simulink model "Water_Supply_Network_AMONG_US"  (R2024a)
settings: Solver=VariableStepAuto  StartTime=0  StopTime=10  RelTol=1e3
model workspace (MAT data in the model file):
  a = [3 8 5 5 2 7 2 5]
  c = [100 100 100 100 100 100 100 100]
  c_init = [50 50 50 0 0 0 0 0]
  d = [2 0.5 4 3 4 5 7 4]
  f = [0.4 0.6 0.2 1 0.4 0.1 0.9 0.6]
  p = [15 20 5 7 3 5 5]
settings Model: Creator=Anna  LastModifiedBy=eveli

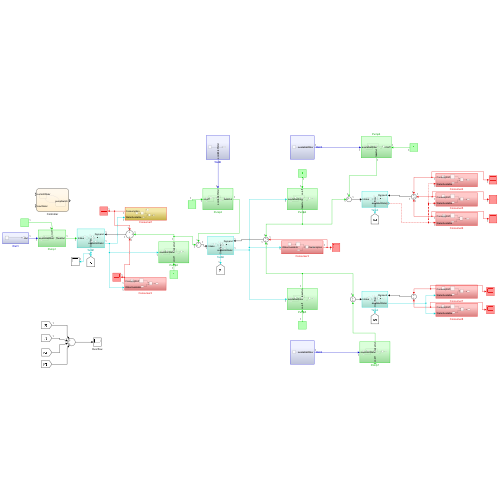
[thumbnail: Simulink's stored preview of the top-level diagram]
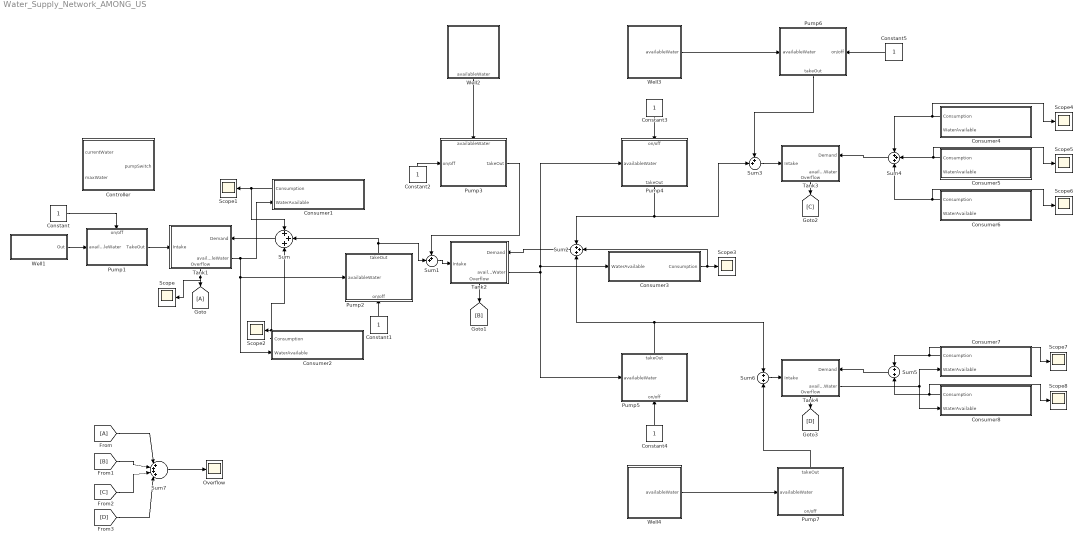
== system Water_Supply_Network_AMONG_US ==
  Constant{,1..5} (6 alike) : Constant  OutDataTypeStr=boolean
  Consumer1 : Subsystem
      settings: PortSchema="{\"entries\":[{\"content\":{\"sides\":[{\"content\":{\"connectorIds\":[\"Out1\",\"In1\"]},\"type\":\"ConnectorPlacement.EquallySpacedRectSide\",\"uuid\":\"64b5a97a-4244-4f26-899d-15714f2aa8f6\"},{\"content\":{\"side\":\"RIGHT\"},\"type\":\"ConnectorPlacement.EquallySpacedRectSide\",\"uuid\":\"d3b45f67-9c9d-4eef-86a5-95557b8542c4\"},{\"content\":{\"side\":\"TOP\"},\"type\":\"ConnectorPlacement.EquallySpacedRectSide\",\"uuid\":\"2b7281c0-f61f-45e3-808b-a4fd1d62cbbb\"}]},\"type\":\"ConnectorPlacement.EquallySpacedConnector\",\"uuid\":\"1937d4df-e955-4a14-a18e-eb0cc3956b4d\"}],\"packageUris\":[\"http://schema.mathworks.com/mf0/Connector/R2020b\"],\"version\":\"1.0\"}"
  Consumer2 : Subsystem
      settings: PortSchema="{\"entries\":[{\"content\":{\"sides\":[{\"content\":{\"connectorIds\":[\"Out1\",\"In1\"]},\"type\":\"ConnectorPlacement.EquallySpacedRectSide\",\"uuid\":\"64b5a97a-4244-4f26-899d-15714f2aa8f6\"},{\"content\":{\"side\":\"RIGHT\"},\"type\":\"ConnectorPlacement.EquallySpacedRectSide\",\"uuid\":\"d3b45f67-9c9d-4eef-86a5-95557b8542c4\"},{\"content\":{\"side\":\"TOP\"},\"type\":\"ConnectorPlacement.EquallySpacedRectSide\",\"uuid\":\"2b7281c0-f61f-45e3-808b-a4fd1d62cbbb\"}]},\"type\":\"ConnectorPlacement.EquallySpacedConnector\",\"uuid\":\"1937d4df-e955-4a14-a18e-eb0cc3956b4d\"}],\"packageUris\":[\"http://schema.mathworks.com/mf0/Connector/R2020b\"],\"version\":\"1.0\"}"
  Consumer3 : Subsystem
  Consumer4 : Subsystem
      settings: PortSchema="{\"entries\":[{\"content\":{\"sides\":[{\"content\":{\"connectorIds\":[\"Out1\",\"In1\"]},\"type\":\"ConnectorPlacement.EquallySpacedRectSide\",\"uuid\":\"64b5a97a-4244-4f26-899d-15714f2aa8f6\"},{\"content\":{\"side\":\"RIGHT\"},\"type\":\"ConnectorPlacement.EquallySpacedRectSide\",\"uuid\":\"d3b45f67-9c9d-4eef-86a5-95557b8542c4\"},{\"content\":{\"side\":\"TOP\"},\"type\":\"ConnectorPlacement.EquallySpacedRectSide\",\"uuid\":\"2b7281c0-f61f-45e3-808b-a4fd1d62cbbb\"}]},\"type\":\"ConnectorPlacement.EquallySpacedConnector\",\"uuid\":\"1937d4df-e955-4a14-a18e-eb0cc3956b4d\"}],\"packageUris\":[\"http://schema.mathworks.com/mf0/Connector/R2020b\"],\"version\":\"1.0\"}"
  Consumer5 : Subsystem
      settings: PortSchema="{\"entries\":[{\"content\":{\"sides\":[{\"content\":{\"connectorIds\":[\"Out1\",\"In1\"]},\"type\":\"ConnectorPlacement.EquallySpacedRectSide\",\"uuid\":\"64b5a97a-4244-4f26-899d-15714f2aa8f6\"},{\"content\":{\"side\":\"RIGHT\"},\"type\":\"ConnectorPlacement.EquallySpacedRectSide\",\"uuid\":\"d3b45f67-9c9d-4eef-86a5-95557b8542c4\"},{\"content\":{\"side\":\"TOP\"},\"type\":\"ConnectorPlacement.EquallySpacedRectSide\",\"uuid\":\"2b7281c0-f61f-45e3-808b-a4fd1d62cbbb\"}]},\"type\":\"ConnectorPlacement.EquallySpacedConnector\",\"uuid\":\"1937d4df-e955-4a14-a18e-eb0cc3956b4d\"}],\"packageUris\":[\"http://schema.mathworks.com/mf0/Connector/R2020b\"],\"version\":\"1.0\"}"
  Consumer6 : Subsystem
      settings: PortSchema="{\"entries\":[{\"content\":{\"sides\":[{\"content\":{\"connectorIds\":[\"Out1\",\"In1\"]},\"type\":\"ConnectorPlacement.EquallySpacedRectSide\",\"uuid\":\"64b5a97a-4244-4f26-899d-15714f2aa8f6\"},{\"content\":{\"side\":\"RIGHT\"},\"type\":\"ConnectorPlacement.EquallySpacedRectSide\",\"uuid\":\"d3b45f67-9c9d-4eef-86a5-95557b8542c4\"},{\"content\":{\"side\":\"TOP\"},\"type\":\"ConnectorPlacement.EquallySpacedRectSide\",\"uuid\":\"2b7281c0-f61f-45e3-808b-a4fd1d62cbbb\"}]},\"type\":\"ConnectorPlacement.EquallySpacedConnector\",\"uuid\":\"1937d4df-e955-4a14-a18e-eb0cc3956b4d\"}],\"packageUris\":[\"http://schema.mathworks.com/mf0/Connector/R2020b\"],\"version\":\"1.0\"}"
  Consumer7 : Subsystem
      settings: PortSchema="{\"entries\":[{\"content\":{\"sides\":[{\"content\":{\"connectorIds\":[\"Out1\",\"In1\"]},\"type\":\"ConnectorPlacement.EquallySpacedRectSide\",\"uuid\":\"64b5a97a-4244-4f26-899d-15714f2aa8f6\"},{\"content\":{\"side\":\"RIGHT\"},\"type\":\"ConnectorPlacement.EquallySpacedRectSide\",\"uuid\":\"d3b45f67-9c9d-4eef-86a5-95557b8542c4\"},{\"content\":{\"side\":\"TOP\"},\"type\":\"ConnectorPlacement.EquallySpacedRectSide\",\"uuid\":\"2b7281c0-f61f-45e3-808b-a4fd1d62cbbb\"}]},\"type\":\"ConnectorPlacement.EquallySpacedConnector\",\"uuid\":\"1937d4df-e955-4a14-a18e-eb0cc3956b4d\"}],\"packageUris\":[\"http://schema.mathworks.com/mf0/Connector/R2020b\"],\"version\":\"1.0\"}"
  Consumer8 : Subsystem
      settings: PortSchema="{\"entries\":[{\"content\":{\"sides\":[{\"content\":{\"connectorIds\":[\"Out1\",\"In1\"]},\"type\":\"ConnectorPlacement.EquallySpacedRectSide\",\"uuid\":\"64b5a97a-4244-4f26-899d-15714f2aa8f6\"},{\"content\":{\"side\":\"RIGHT\"},\"type\":\"ConnectorPlacement.EquallySpacedRectSide\",\"uuid\":\"d3b45f67-9c9d-4eef-86a5-95557b8542c4\"},{\"content\":{\"side\":\"TOP\"},\"type\":\"ConnectorPlacement.EquallySpacedRectSide\",\"uuid\":\"2b7281c0-f61f-45e3-808b-a4fd1d62cbbb\"}]},\"type\":\"ConnectorPlacement.EquallySpacedConnector\",\"uuid\":\"1937d4df-e955-4a14-a18e-eb0cc3956b4d\"}],\"packageUris\":[\"http://schema.mathworks.com/mf0/Connector/R2020b\"],\"version\":\"1.0\"}"
  Controller : Stateflow chart  TreatAsAtomicUnit=on
  From : From
  Goto : Goto
  Overflow : Scope
  Pump1 : Subsystem
      settings: PortSchema="{\"entries\":[{\"content\":{\"sides\":[{\"content\":{\"connectorIds\":[\"In1\"]},\"type\":\"ConnectorPlacement.EquallySpacedRectSide\",\"uuid\":\"19044534-5fed-425e-9b28-cfa8ce8c2d07\"},{\"content\":{\"connectorIds\":[\"Out1\"],\"side\":\"RIGHT\"},\"type\":\"ConnectorPlacement.EquallySpacedRectSide\",\"uuid\":\"25083535-857b-4aa6-b643-c29d52fd8b89\"},{\"content\":{\"connectorIds\":[\"In2\"],\"side\":\"TOP\"},\"type\":\"ConnectorPlacement.EquallySpacedRectSide\",\"uuid\":\"599575d0-15e5-44fc-9209-be917a93ad07\"}]},\"type\":\"ConnectorPlacement.EquallySpacedConnector\",\"uuid\":\"7a1b4f14-afb7-42e2-aa80-653c0fb5067f\"}],\"packageUris\":[\"http://schema.mathworks.com/mf0/Connector/R2020b\"],\"version\":\"1.0\"}"
  Pump2 : Subsystem
      settings: PortSchema="{\"entries\":[{\"content\":{\"sides\":[{\"content\":{\"connectorIds\":[\"In1\"]},\"type\":\"ConnectorPlacement.EquallySpacedRectSide\",\"uuid\":\"19044534-5fed-425e-9b28-cfa8ce8c2d07\"},{\"content\":{\"side\":\"RIGHT\"},\"type\":\"ConnectorPlacement.EquallySpacedRectSide\",\"uuid\":\"25083535-857b-4aa6-b643-c29d52fd8b89\"},{\"content\":{\"connectorIds\":[\"Out1\"],\"side\":\"TOP\"},\"type\":\"ConnectorPlacement.EquallySpacedRectSide\",\"uuid\":\"599575d0-15e5-44fc-9209-be917a93ad07\"},{\"content\":{\"connectorIds\":[\"In2\"],\"side\":\"BOTTOM\"},\"type\":\"ConnectorPlacement.EquallySpacedRectSide\",\"uuid\":\"52860d2e-e532-4b54-b4dc-ac60bb6223b5\"}]},\"type\":\"ConnectorPlacement.EquallySpacedConnector\",\"uuid\":\"7a1b4f14-afb7-42e2-aa80-653c0fb5067f\"}],\"packageUris\":[\"http://schema.mathworks.com/mf0/Connector/R2020b\"],\"version\":\"1.0\"}"
  Pump3 : Subsystem
      settings: PortSchema="{\"entries\":[{\"content\":{\"sides\":[{\"content\":{\"connectorIds\":[\"In1\"]},\"type\":\"ConnectorPlacement.EquallySpacedRectSide\",\"uuid\":\"19044534-5fed-425e-9b28-cfa8ce8c2d07\"},{\"content\":{\"connectorIds\":[\"Out1\"],\"side\":\"RIGHT\"},\"type\":\"ConnectorPlacement.EquallySpacedRectSide\",\"uuid\":\"25083535-857b-4aa6-b643-c29d52fd8b89\"},{\"content\":{\"connectorIds\":[\"In2\"],\"side\":\"TOP\"},\"type\":\"ConnectorPlacement.EquallySpacedRectSide\",\"uuid\":\"599575d0-15e5-44fc-9209-be917a93ad07\"},{\"content\":{\"side\":\"BOTTOM\"},\"type\":\"ConnectorPlacement.EquallySpacedRectSide\",\"uuid\":\"52860d2e-e532-4b54-b4dc-ac60bb6223b5\"}]},\"type\":\"ConnectorPlacement.EquallySpacedConnector\",\"uuid\":\"7a1b4f14-afb7-42e2-aa80-653c0fb5067f\"}],\"packageUris\":[\"http://schema.mathworks.com/mf0/Connector/R2020b\"],\"version\":\"1.0\"}"
  Pump4 : Subsystem
      settings: PortSchema="{\"entries\":[{\"content\":{\"sides\":[{\"content\":{\"connectorIds\":[\"In1\"]},\"type\":\"ConnectorPlacement.EquallySpacedRectSide\",\"uuid\":\"19044534-5fed-425e-9b28-cfa8ce8c2d07\"},{\"content\":{\"side\":\"RIGHT\"},\"type\":\"ConnectorPlacement.EquallySpacedRectSide\",\"uuid\":\"25083535-857b-4aa6-b643-c29d52fd8b89\"},{\"content\":{\"connectorIds\":[\"In2\"],\"side\":\"TOP\"},\"type\":\"ConnectorPlacement.EquallySpacedRectSide\",\"uuid\":\"599575d0-15e5-44fc-9209-be917a93ad07\"},{\"content\":{\"connectorIds\":[\"Out1\"],\"side\":\"BOTTOM\"},\"type\":\"ConnectorPlacement.EquallySpacedRectSide\",\"uuid\":\"52860d2e-e532-4b54-b4dc-ac60bb6223b5\"}]},\"type\":\"ConnectorPlacement.EquallySpacedConnector\",\"uuid\":\"7a1b4f14-afb7-42e2-aa80-653c0fb5067f\"}],\"packageUris\":[\"http://schema.mathworks.com/mf0/Connector/R2020b\"],\"version\":\"1.0\"}"
  Pump5 : Subsystem
      settings: PortSchema="{\"entries\":[{\"content\":{\"sides\":[{\"content\":{\"connectorIds\":[\"In1\"]},\"type\":\"ConnectorPlacement.EquallySpacedRectSide\",\"uuid\":\"19044534-5fed-425e-9b28-cfa8ce8c2d07\"},{\"content\":{\"side\":\"RIGHT\"},\"type\":\"ConnectorPlacement.EquallySpacedRectSide\",\"uuid\":\"25083535-857b-4aa6-b643-c29d52fd8b89\"},{\"content\":{\"connectorIds\":[\"Out1\"],\"side\":\"TOP\"},\"type\":\"ConnectorPlacement.EquallySpacedRectSide\",\"uuid\":\"599575d0-15e5-44fc-9209-be917a93ad07\"},{\"content\":{\"connectorIds\":[\"In2\"],\"side\":\"BOTTOM\"},\"type\":\"ConnectorPlacement.EquallySpacedRectSide\",\"uuid\":\"52860d2e-e532-4b54-b4dc-ac60bb6223b5\"}]},\"type\":\"ConnectorPlacement.EquallySpacedConnector\",\"uuid\":\"7a1b4f14-afb7-42e2-aa80-653c0fb5067f\"}],\"packageUris\":[\"http://schema.mathworks.com/mf0/Connector/R2020b\"],\"version\":\"1.0\"}"
  Pump6 : Subsystem
      settings: PortSchema="{\"entries\":[{\"content\":{\"sides\":[{\"content\":{\"connectorIds\":[\"In1\"]},\"type\":\"ConnectorPlacement.EquallySpacedRectSide\",\"uuid\":\"19044534-5fed-425e-9b28-cfa8ce8c2d07\"},{\"content\":{\"connectorIds\":[\"In2\"],\"side\":\"RIGHT\"},\"type\":\"ConnectorPlacement.EquallySpacedRectSide\",\"uuid\":\"25083535-857b-4aa6-b643-c29d52fd8b89\"},{\"content\":{\"connectorIds\":[\"Out1\"],\"side\":\"TOP\"},\"type\":\"ConnectorPlacement.EquallySpacedRectSide\",\"uuid\":\"599575d0-15e5-44fc-9209-be917a93ad07\"},{\"content\":{\"side\":\"BOTTOM\"},\"type\":\"ConnectorPlacement.EquallySpacedRectSide\",\"uuid\":\"52860d2e-e532-4b54-b4dc-ac60bb6223b5\"}]},\"type\":\"ConnectorPlacement.EquallySpacedConnector\",\"uuid\":\"7a1b4f14-afb7-42e2-aa80-653c0fb5067f\"}],\"packageUris\":[\"http://schema.mathworks.com/mf0/Connector/R2020b\"],\"version\":\"1.0\"}"
  Pump7 : Subsystem
      settings: PortSchema="{\"entries\":[{\"content\":{\"sides\":[{\"content\":{\"connectorIds\":[\"In1\"]},\"type\":\"ConnectorPlacement.EquallySpacedRectSide\",\"uuid\":\"19044534-5fed-425e-9b28-cfa8ce8c2d07\"},{\"content\":{\"side\":\"RIGHT\"},\"type\":\"ConnectorPlacement.EquallySpacedRectSide\",\"uuid\":\"25083535-857b-4aa6-b643-c29d52fd8b89\"},{\"content\":{\"connectorIds\":[\"Out1\"],\"side\":\"TOP\"},\"type\":\"ConnectorPlacement.EquallySpacedRectSide\",\"uuid\":\"599575d0-15e5-44fc-9209-be917a93ad07\"},{\"content\":{\"connectorIds\":[\"In2\"],\"side\":\"BOTTOM\"},\"type\":\"ConnectorPlacement.EquallySpacedRectSide\",\"uuid\":\"52860d2e-e532-4b54-b4dc-ac60bb6223b5\"}]},\"type\":\"ConnectorPlacement.EquallySpacedConnector\",\"uuid\":\"7a1b4f14-afb7-42e2-aa80-653c0fb5067f\"}],\"packageUris\":[\"http://schema.mathworks.com/mf0/Connector/R2020b\"],\"version\":\"1.0\"}"
  Scope{,1..8} (9 alike) : Scope
  Sum : Sum  Inputs=+++
  Sum1 : Sum  Inputs=++|
  Sum2 : Sum  Inputs=+++
  Sum3 : Sum  Inputs=++|
  Sum4 : Sum  Inputs=+++
  Sum5 : Sum
  Sum6 : Sum
  Sum7 : Sum  Inputs=|++++|
  Tank1 : Subsystem
      settings: PortSchema="{\"entries\":[{\"content\":{\"sides\":[{\"content\":{\"connectorIds\":[\"In1\"]},\"type\":\"ConnectorPlacement.EquallySpacedRectSide\",\"uuid\":\"19044534-5fed-425e-9b28-cfa8ce8c2d07\"},{\"content\":{\"connectorIds\":[\"In2\",\"Out1\"],\"side\":\"RIGHT\"},\"type\":\"ConnectorPlacement.EquallySpacedRectSide\",\"uuid\":\"25083535-857b-4aa6-b643-c29d52fd8b89\"},{\"content\":{\"side\":\"TOP\"},\"type\":\"ConnectorPlacement.EquallySpacedRectSide\",\"uuid\":\"599575d0-15e5-44fc-9209-be917a93ad07\"},{\"content\":{\"connectorIds\":[\"Out2\"],\"side\":\"BOTTOM\"},\"type\":\"ConnectorPlacement.EquallySpacedRectSide\",\"uuid\":\"799f4d24-f4f0-4738-a8a2-f0c8281d36dc\"}]},\"type\":\"ConnectorPlacement.EquallySpacedConnector\",\"uuid\":\"7a1b4f14-afb7-42e2-aa80-653c0fb5067f\"}],\"packageUris\":[\"http://schema.mathworks.com/mf0/Connector/R2020b\"],\"version\":\"1.0\"}"
  Tank2 : Subsystem
      settings: PortSchema="{\"entries\":[{\"content\":{\"sides\":[{\"content\":{\"connectorIds\":[\"In1\"]},\"type\":\"ConnectorPlacement.EquallySpacedRectSide\",\"uuid\":\"6394a9ac-99af-493e-a9a9-7a018208ef50\"},{\"content\":{\"connectorIds\":[\"In2\",\"Out1\"],\"side\":\"RIGHT\"},\"type\":\"ConnectorPlacement.EquallySpacedRectSide\",\"uuid\":\"612acb37-252a-4856-85fd-674ec3c616cc\"},{\"content\":{\"side\":\"TOP\"},\"type\":\"ConnectorPlacement.EquallySpacedRectSide\",\"uuid\":\"1047c534-4c6b-441e-a3b9-f8dd3232279a\"},{\"content\":{\"connectorIds\":[\"Out2\"],\"side\":\"BOTTOM\"},\"type\":\"ConnectorPlacement.EquallySpacedRectSide\",\"uuid\":\"42885eae-c582-4672-94f7-20fc857473a2\"}]},\"type\":\"ConnectorPlacement.EquallySpacedConnector\",\"uuid\":\"ec171fb9-b944-410c-8959-17a79b80883c\"}],\"packageUris\":[\"http://schema.mathworks.com/mf0/Connector/R2020b\"],\"version\":\"1.0\"}"
  Tank3 : Subsystem
      settings: PortSchema="{\"entries\":[{\"content\":{\"sides\":[{\"content\":{\"connectorIds\":[\"In1\"]},\"type\":\"ConnectorPlacement.EquallySpacedRectSide\",\"uuid\":\"6394a9ac-99af-493e-a9a9-7a018208ef50\"},{\"content\":{\"connectorIds\":[\"In2\",\"Out1\"],\"side\":\"RIGHT\"},\"type\":\"ConnectorPlacement.EquallySpacedRectSide\",\"uuid\":\"612acb37-252a-4856-85fd-674ec3c616cc\"},{\"content\":{\"side\":\"TOP\"},\"type\":\"ConnectorPlacement.EquallySpacedRectSide\",\"uuid\":\"1047c534-4c6b-441e-a3b9-f8dd3232279a\"},{\"content\":{\"connectorIds\":[\"Out2\"],\"side\":\"BOTTOM\"},\"type\":\"ConnectorPlacement.EquallySpacedRectSide\",\"uuid\":\"9e3905b0-9668-48de-b5ad-5e7359606e89\"}]},\"type\":\"ConnectorPlacement.EquallySpacedConnector\",\"uuid\":\"ec171fb9-b944-410c-8959-17a79b80883c\"}],\"packageUris\":[\"http://schema.mathworks.com/mf0/Connector/R2020b\"],\"version\":\"1.0\"}"
  Tank4 : Subsystem
      settings: PortSchema="{\"entries\":[{\"content\":{\"sides\":[{\"content\":{\"connectorIds\":[\"In1\"]},\"type\":\"ConnectorPlacement.EquallySpacedRectSide\",\"uuid\":\"6394a9ac-99af-493e-a9a9-7a018208ef50\"},{\"content\":{\"connectorIds\":[\"In2\",\"Out1\"],\"side\":\"RIGHT\"},\"type\":\"ConnectorPlacement.EquallySpacedRectSide\",\"uuid\":\"612acb37-252a-4856-85fd-674ec3c616cc\"},{\"content\":{\"side\":\"TOP\"},\"type\":\"ConnectorPlacement.EquallySpacedRectSide\",\"uuid\":\"1047c534-4c6b-441e-a3b9-f8dd3232279a\"},{\"content\":{\"connectorIds\":[\"Out2\"],\"side\":\"BOTTOM\"},\"type\":\"ConnectorPlacement.EquallySpacedRectSide\",\"uuid\":\"74ff9e79-0f60-4283-af2e-661939d7d190\"}]},\"type\":\"ConnectorPlacement.EquallySpacedConnector\",\"uuid\":\"ec171fb9-b944-410c-8959-17a79b80883c\"}],\"packageUris\":[\"http://schema.mathworks.com/mf0/Connector/R2020b\"],\"version\":\"1.0\"}"
  Well1 : Subsystem
  Well2 : Subsystem
      settings: PortSchema="{\"entries\":[{\"content\":{\"sides\":[{\"content\":{},\"type\":\"ConnectorPlacement.EquallySpacedRectSide\",\"uuid\":\"4390e0f2-eeab-466a-9818-e6d81af1fb71\"},{\"content\":{\"side\":\"RIGHT\"},\"type\":\"ConnectorPlacement.EquallySpacedRectSide\",\"uuid\":\"9d0fea14-12b9-47ed-a07e-c6f020298b95\"},{\"content\":{\"side\":\"TOP\"},\"type\":\"ConnectorPlacement.EquallySpacedRectSide\",\"uuid\":\"70893623-e241-4278-8eee-4ec70d637e6e\"},{\"content\":{\"connectorIds\":[\"Out1\"],\"side\":\"BOTTOM\"},\"type\":\"ConnectorPlacement.EquallySpacedRectSide\",\"uuid\":\"3974d751-8f92-4944-8346-f968cf92cbe1\"}]},\"type\":\"ConnectorPlacement.EquallySpacedConnector\",\"uuid\":\"1eb64d0b-eb34-4a37-b2c5-2df08b99f7d9\"}],\"packageUris\":[\"http://schema.mathworks.com/mf0/Connector/R2020b\"],\"version\":\"1.0\"}"
  Well3 : Subsystem
      settings: PortSchema="{\"entries\":[{\"content\":{\"sides\":[{\"content\":{},\"type\":\"ConnectorPlacement.EquallySpacedRectSide\",\"uuid\":\"4390e0f2-eeab-466a-9818-e6d81af1fb71\"},{\"content\":{\"side\":\"RIGHT\"},\"type\":\"ConnectorPlacement.EquallySpacedRectSide\",\"uuid\":\"9d0fea14-12b9-47ed-a07e-c6f020298b95\"},{\"content\":{\"side\":\"TOP\"},\"type\":\"ConnectorPlacement.EquallySpacedRectSide\",\"uuid\":\"70893623-e241-4278-8eee-4ec70d637e6e\"},{\"content\":{\"connectorIds\":[\"Out1\"],\"side\":\"BOTTOM\"},\"type\":\"ConnectorPlacement.EquallySpacedRectSide\",\"uuid\":\"3974d751-8f92-4944-8346-f968cf92cbe1\"}]},\"type\":\"ConnectorPlacement.EquallySpacedConnector\",\"uuid\":\"1eb64d0b-eb34-4a37-b2c5-2df08b99f7d9\"}],\"packageUris\":[\"http://schema.mathworks.com/mf0/Connector/R2020b\"],\"version\":\"1.0\"}"
  Well4 : Subsystem
      settings: PortSchema="{\"entries\":[{\"content\":{\"sides\":[{\"content\":{},\"type\":\"ConnectorPlacement.EquallySpacedRectSide\",\"uuid\":\"4390e0f2-eeab-466a-9818-e6d81af1fb71\"},{\"content\":{\"side\":\"RIGHT\"},\"type\":\"ConnectorPlacement.EquallySpacedRectSide\",\"uuid\":\"9d0fea14-12b9-47ed-a07e-c6f020298b95\"},{\"content\":{\"side\":\"TOP\"},\"type\":\"ConnectorPlacement.EquallySpacedRectSide\",\"uuid\":\"70893623-e241-4278-8eee-4ec70d637e6e\"},{\"content\":{\"connectorIds\":[\"Out1\"],\"side\":\"BOTTOM\"},\"type\":\"ConnectorPlacement.EquallySpacedRectSide\",\"uuid\":\"3974d751-8f92-4944-8346-f968cf92cbe1\"}]},\"type\":\"ConnectorPlacement.EquallySpacedConnector\",\"uuid\":\"1eb64d0b-eb34-4a37-b2c5-2df08b99f7d9\"}],\"packageUris\":[\"http://schema.mathworks.com/mf0/Connector/R2020b\"],\"version\":\"1.0\"}"
  wires:
  Constant/1 -> Pump1/2(on/off)
  Pump1/1(TakeOut) -> Tank1/1(Intake)
  Well1/1(Out) -> Pump1/1(availableWater)
  Tank1/1(availableWater) -> Consumer1/1(WaterAvailable), Consumer2/1(WaterAvailable), Pump2/1(availableWater)
  Consumer1/1(Consumption) -> Sum/1, Scope1/1
  Consumer2/1(Consumption) -> Sum/3, Scope2/1
  Sum/1 -> Tank1/2(Demand)
  Pump2/1(takeOut) -> Sum1/2, Sum/2
  Constant1/1 -> Pump2/2(on/off)
  Constant2/1 -> Pump3/1(on/off)
  Well2/1(availableWater) -> Pump3/2(availableWater)
  Sum1/1 -> Tank2/1(Intake)
  Pump3/1(takeOut) -> Sum1/1
  Constant3/1 -> Pump4/2(on/off)
  Constant4/1 -> Pump5/2(on/off)
  Tank2/1(availableWater) -> Pump4/1(availableWater), Consumer3/1(WaterAvailable), Pump5/1(availableWater)
  Consumer3/1(Consumption) -> Sum2/2, Scope3/1
  Pump4/1(takeOut) -> Sum3/2, Sum2/1
  Pump5/1(takeOut) -> Sum6/1, Sum2/3
  Constant5/1 -> Pump6/1(on/off)
  Pump6/1(takeOut) -> Sum3/1
  Sum3/1 -> Tank3/1(Intake)
  Well3/1(availableWater) -> Pump6/2(availableWater)
  Sum4/1 -> Tank3/2(Demand)
  Consumer4/1(Consumption) -> Scope4/1, Sum4/1
  Consumer5/1(Consumption) -> Scope5/1, Sum4/2
  Consumer6/1(Consumption) -> Scope6/1, Sum4/3
  ? -> Consumer4/1(WaterAvailable), Consumer5/1(WaterAvailable), Consumer6/1(WaterAvailable)
  Consumer8/1(Consumption) -> Scope8/1, Sum5/2
  Consumer7/1(Consumption) -> Scope7/1, Sum5/1
  Sum5/1 -> Tank4/2(Demand)
  Tank4/1(availableWater) -> Consumer8/1(WaterAvailable), Consumer7/1(WaterAvailable)
  Well4/1(availableWater) -> Pump7/1(availableWater)
  Pump7/1(takeOut) -> Sum6/2
  Sum6/1 -> Tank4/1(Intake)
  Sum2/1 -> Tank2/2(Demand)
  Tank1/2(Overflow) -> Scope/1, Goto/1
  Tank2/2(Overflow) -> [B]
  Tank3/2(Overflow) -> [C]
  Tank4/2(Overflow) -> [D]
  From/1 -> Sum7/1
  [B] -> Sum7/2
  [C] -> Sum7/3
  [D] -> Sum7/4
  Sum7/1 -> Overflow/1

== system Water_Supply_Network_AMONG_US/Consumer1 ==
  WaterAvailable : Inport
  Min : MinMax  Inputs=2
  Scope : Scope
  Sine Wave : Sin  Amplitude=a(1)  Bias=a(1)  Frequency=f(1)  SampleTime=0
  Transport Delay : TransportDelay  DelayTime=d(1)  InitialOutput=a(1)
  Consumption : Outport
  wires:
  WaterAvailable/1 -> Min/2
  Min/1 -> Consumption/1
  Transport Delay/1 -> Scope/1, Min/1
  Sine Wave/1 -> Transport Delay/1

== system Water_Supply_Network_AMONG_US/Consumer2 ==
  WaterAvailable : Inport
  Min : MinMax  Inputs=2
  Sine Wave : Sin  Amplitude=a(2)  Bias=a(2)  Frequency=f(2)  SampleTime=0
  Transport Delay : TransportDelay  DelayTime=d(2)  InitialOutput=a(2)
  Consumption : Outport
  wires:
  Sine Wave/1 -> Transport Delay/1
  WaterAvailable/1 -> Min/2
  Min/1 -> Consumption/1
  Transport Delay/1 -> Min/1

== system Water_Supply_Network_AMONG_US/Consumer3 ==
  WaterAvailable : Inport
  Min : MinMax  Inputs=2
  Sine Wave : Sin  Amplitude=a(3)  Bias=a(3)  Frequency=f(3)  SampleTime=0
  Transport Delay : TransportDelay  DelayTime=d(3)  InitialOutput=a(3)
  Consumption : Outport
  wires:
  Sine Wave/1 -> Transport Delay/1
  WaterAvailable/1 -> Min/2
  Min/1 -> Consumption/1
  Transport Delay/1 -> Min/1

== system Water_Supply_Network_AMONG_US/Consumer4 ==
  WaterAvailable : Inport
  Min : MinMax  Inputs=2
  Sine Wave : Sin  Amplitude=a(4)  Bias=a(4)  Frequency=f(4)  SampleTime=0
  Transport Delay : TransportDelay  DelayTime=d(4)  InitialOutput=a(4)
  Consumption : Outport
  wires:
  Sine Wave/1 -> Transport Delay/1
  WaterAvailable/1 -> Min/2
  Min/1 -> Consumption/1
  Transport Delay/1 -> Min/1

== system Water_Supply_Network_AMONG_US/Consumer5 ==
  WaterAvailable : Inport
  Min : MinMax  Inputs=2
  Sine Wave : Sin  Amplitude=a(5)  Bias=a(5)  Frequency=f(5)  SampleTime=0
  Transport Delay : TransportDelay  DelayTime=d(5)  InitialOutput=a(5)
  Consumption : Outport
  wires:
  Sine Wave/1 -> Transport Delay/1
  WaterAvailable/1 -> Min/2
  Min/1 -> Consumption/1
  Transport Delay/1 -> Min/1

== system Water_Supply_Network_AMONG_US/Consumer6 ==
  WaterAvailable : Inport
  Min : MinMax  Inputs=2
  Sine Wave : Sin  Amplitude=a(6)  Bias=a(6)  Frequency=f(6)  SampleTime=0
  Transport Delay : TransportDelay  DelayTime=d(6)  InitialOutput=a(6)
  Consumption : Outport
  wires:
  Sine Wave/1 -> Transport Delay/1
  WaterAvailable/1 -> Min/2
  Min/1 -> Consumption/1
  Transport Delay/1 -> Min/1

== system Water_Supply_Network_AMONG_US/Consumer7 ==
  WaterAvailable : Inport
  Min : MinMax  Inputs=2
  Sine Wave : Sin  Amplitude=a(7)  Bias=a(7)  Frequency=f(7)  SampleTime=0
  Transport Delay : TransportDelay  DelayTime=d(7)  InitialOutput=a(7)
  Consumption : Outport
  wires:
  Sine Wave/1 -> Transport Delay/1
  WaterAvailable/1 -> Min/2
  Min/1 -> Consumption/1
  Transport Delay/1 -> Min/1

== system Water_Supply_Network_AMONG_US/Consumer8 ==
  WaterAvailable : Inport
  Min : MinMax  Inputs=2
  Sine Wave : Sin  Amplitude=a(8)  Bias=a(8)  Frequency=f(8)  SampleTime=0
  Transport Delay : TransportDelay  DelayTime=d(8)  InitialOutput=a(8)
  Consumption : Outport
  wires:
  Sine Wave/1 -> Transport Delay/1
  WaterAvailable/1 -> Min/2
  Min/1 -> Consumption/1
  Transport Delay/1 -> Min/1

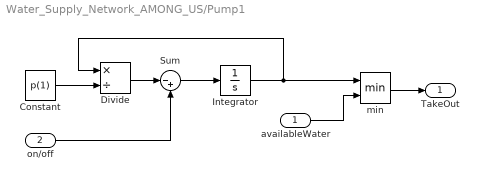
== system Water_Supply_Network_AMONG_US/Pump1 ==
  availableWater : Inport
  on/off : Inport  Port=2  OutDataTypeStr=boolean
  Constant : Constant  Value=p(1)
  Divide : Product  Inputs=*/
  Integrator : Integrator
  Sum : Sum  Inputs=|-+
  min : MinMax  Inputs=2
  TakeOut : Outport
  wires:
  on/off/1 -> Sum/2
  Sum/1 -> Integrator/1
  Integrator/1 -> Divide/1, min/1
  Constant/1 -> Divide/2
  Divide/1 -> Sum/1
  availableWater/1 -> min/2
  min/1 -> TakeOut/1

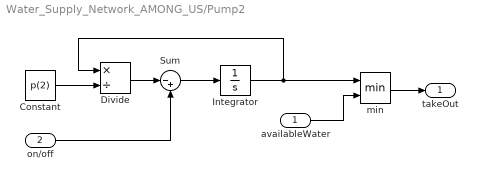
== system Water_Supply_Network_AMONG_US/Pump2 ==
  availableWater : Inport
  on/off : Inport  Port=2  OutDataTypeStr=boolean
  Constant : Constant  Value=p(2)
  Divide : Product  Inputs=*/
  Integrator : Integrator
  Sum : Sum  Inputs=|-+
  min : MinMax  Inputs=2
  takeOut : Outport
  wires:
  on/off/1 -> Sum/2
  Sum/1 -> Integrator/1
  Integrator/1 -> Divide/1, min/1
  Constant/1 -> Divide/2
  Divide/1 -> Sum/1
  availableWater/1 -> min/2
  min/1 -> takeOut/1

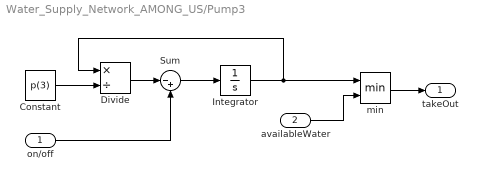
== system Water_Supply_Network_AMONG_US/Pump3 ==
  on/off : Inport  OutDataTypeStr=boolean
  availableWater : Inport  Port=2
  Constant : Constant  Value=p(3)
  Divide : Product  Inputs=*/
  Integrator : Integrator
  Sum : Sum  Inputs=|-+
  min : MinMax  Inputs=2
  takeOut : Outport
  wires:
  on/off/1 -> Sum/2
  Sum/1 -> Integrator/1
  Integrator/1 -> Divide/1, min/1
  Constant/1 -> Divide/2
  Divide/1 -> Sum/1
  availableWater/1 -> min/2
  min/1 -> takeOut/1

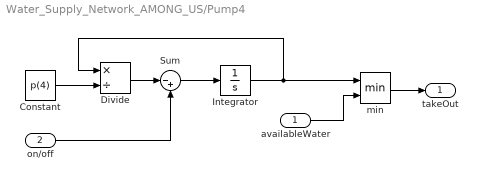
== system Water_Supply_Network_AMONG_US/Pump4 ==
  availableWater : Inport
  on/off : Inport  Port=2  OutDataTypeStr=boolean
  Constant : Constant  Value=p(4)
  Divide : Product  Inputs=*/
  Integrator : Integrator
  Sum : Sum  Inputs=|-+
  min : MinMax  Inputs=2
  takeOut : Outport
  wires:
  on/off/1 -> Sum/2
  Sum/1 -> Integrator/1
  Integrator/1 -> Divide/1, min/1
  Constant/1 -> Divide/2
  Divide/1 -> Sum/1
  availableWater/1 -> min/2
  min/1 -> takeOut/1

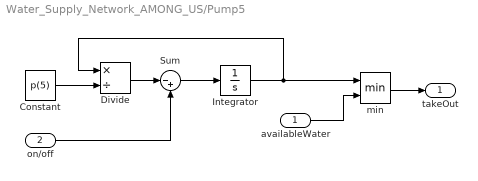
== system Water_Supply_Network_AMONG_US/Pump5 ==
  availableWater : Inport
  on/off : Inport  Port=2  OutDataTypeStr=boolean
  Constant : Constant  Value=p(5)
  Divide : Product  Inputs=*/
  Integrator : Integrator
  Sum : Sum  Inputs=|-+
  min : MinMax  Inputs=2
  takeOut : Outport
  wires:
  on/off/1 -> Sum/2
  Sum/1 -> Integrator/1
  Integrator/1 -> Divide/1, min/1
  Constant/1 -> Divide/2
  Divide/1 -> Sum/1
  availableWater/1 -> min/2
  min/1 -> takeOut/1

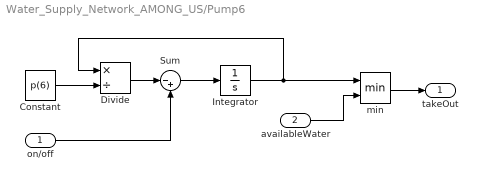
== system Water_Supply_Network_AMONG_US/Pump6 ==
  on/off : Inport  OutDataTypeStr=boolean
  availableWater : Inport  Port=2
  Constant : Constant  Value=p(6)
  Divide : Product  Inputs=*/
  Integrator : Integrator
  Sum : Sum  Inputs=|-+
  min : MinMax  Inputs=2
  takeOut : Outport
  wires:
  on/off/1 -> Sum/2
  Sum/1 -> Integrator/1
  Integrator/1 -> Divide/1, min/1
  Constant/1 -> Divide/2
  Divide/1 -> Sum/1
  availableWater/1 -> min/2
  min/1 -> takeOut/1

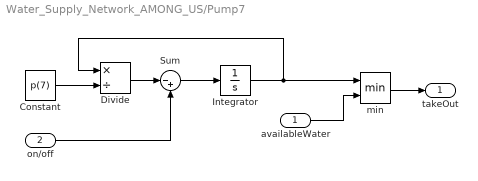
== system Water_Supply_Network_AMONG_US/Pump7 ==
  availableWater : Inport
  on/off : Inport  Port=2  OutDataTypeStr=boolean
  Constant : Constant  Value=p(7)
  Divide : Product  Inputs=*/
  Integrator : Integrator
  Sum : Sum  Inputs=|-+
  min : MinMax  Inputs=2
  takeOut : Outport
  wires:
  on/off/1 -> Sum/2
  Sum/1 -> Integrator/1
  Integrator/1 -> Divide/1, min/1
  Constant/1 -> Divide/2
  Divide/1 -> Sum/1
  availableWater/1 -> min/2
  min/1 -> takeOut/1

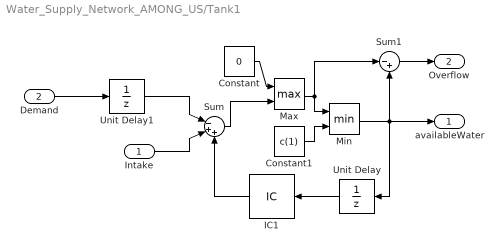
== system Water_Supply_Network_AMONG_US/Tank1 ==
  Intake : Inport
  Demand : Inport  Port=2
  Constant : Constant  Value=0
  Constant1 : Constant  Value=c(1)
  IC1 : InitialCondition  Value=c_init(1)
  Max : MinMax  Function=max  Inputs=2
  Min : MinMax  Inputs=2
  Sum : Sum  Inputs=|-++
  Sum1 : Sum  Inputs=|-+
  Unit Delay : UnitDelay  SampleTime=-1  HasFrameUpgradeWarning=on
  Unit Delay1 : UnitDelay  SampleTime=-1  HasFrameUpgradeWarning=on
  availableWater : Outport
  Overflow : Outport  Port=2
  wires:
  Intake/1 -> Sum/2
  Demand/1 -> Unit Delay1/1
  Sum/1 -> Max/2
  IC1/1 -> Sum/3
  Constant/1 -> Max/1
  Max/1 -> Min/1, Sum1/1
  Constant1/1 -> Min/2
  Min/1 -> Unit Delay/1, availableWater/1, Sum1/2
  Sum1/1 -> Overflow/1
  Unit Delay/1 -> IC1/1
  Unit Delay1/1 -> Sum/1

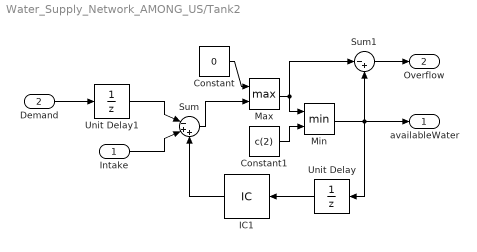
== system Water_Supply_Network_AMONG_US/Tank2 ==
  Intake : Inport
  Demand : Inport  Port=2
  Constant : Constant  Value=0
  Constant1 : Constant  Value=c(2)
  IC1 : InitialCondition  Value=c_init(2)
  Max : MinMax  Function=max  Inputs=2
  Min : MinMax  Inputs=2
  Sum : Sum  Inputs=|-++
  Sum1 : Sum  Inputs=|-+
  Unit Delay : UnitDelay  SampleTime=-1  HasFrameUpgradeWarning=on
  Unit Delay1 : UnitDelay  SampleTime=-1  HasFrameUpgradeWarning=on
  availableWater : Outport
  Overflow : Outport  Port=2
  wires:
  Unit Delay/1 -> IC1/1
  Min/1 -> Unit Delay/1, availableWater/1, Sum1/2
  Constant1/1 -> Min/2
  Sum1/1 -> Overflow/1
  Sum/1 -> Max/2
  Max/1 -> Min/1, Sum1/1
  IC1/1 -> Sum/3
  Intake/1 -> Sum/2
  Constant/1 -> Max/1
  Demand/1 -> Unit Delay1/1
  Unit Delay1/1 -> Sum/1

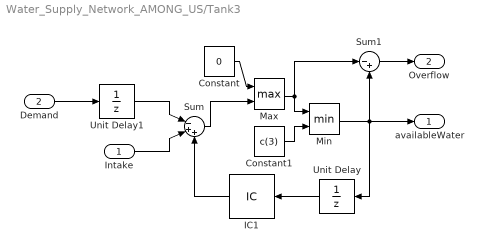
== system Water_Supply_Network_AMONG_US/Tank3 ==
  Intake : Inport
  Demand : Inport  Port=2
  Constant : Constant  Value=0
  Constant1 : Constant  Value=c(3)
  IC1 : InitialCondition  Value=c_init(3)
  Max : MinMax  Function=max  Inputs=2
  Min : MinMax  Inputs=2
  Sum : Sum  Inputs=|-++
  Sum1 : Sum  Inputs=|-+
  Unit Delay : UnitDelay  SampleTime=-1  HasFrameUpgradeWarning=on
  Unit Delay1 : UnitDelay  SampleTime=-1  HasFrameUpgradeWarning=on
  availableWater : Outport
  Overflow : Outport  Port=2
  wires:
  Unit Delay/1 -> IC1/1
  Min/1 -> Unit Delay/1, availableWater/1, Sum1/2
  Constant1/1 -> Min/2
  Sum1/1 -> Overflow/1
  Sum/1 -> Max/2
  Max/1 -> Min/1, Sum1/1
  IC1/1 -> Sum/3
  Intake/1 -> Sum/2
  Constant/1 -> Max/1
  Demand/1 -> Unit Delay1/1
  Unit Delay1/1 -> Sum/1

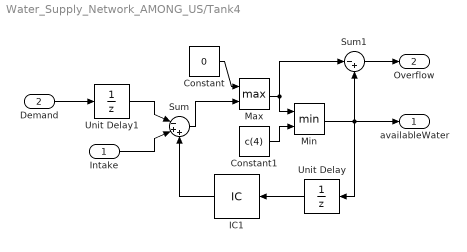
== system Water_Supply_Network_AMONG_US/Tank4 ==
  Intake : Inport
  Demand : Inport  Port=2
  Constant : Constant  Value=0
  Constant1 : Constant  Value=c(4)
  IC1 : InitialCondition  Value=c_init(4)
  Max : MinMax  Function=max  Inputs=2
  Min : MinMax  Inputs=2
  Sum : Sum  Inputs=|-++
  Sum1 : Sum  Inputs=|-+
  Unit Delay : UnitDelay  SampleTime=-1  HasFrameUpgradeWarning=on
  Unit Delay1 : UnitDelay  SampleTime=-1  HasFrameUpgradeWarning=on
  availableWater : Outport
  Overflow : Outport  Port=2
  wires:
  Unit Delay/1 -> IC1/1
  Min/1 -> Unit Delay/1, availableWater/1, Sum1/2
  Constant1/1 -> Min/2
  Sum1/1 -> Overflow/1
  Sum/1 -> Max/2
  Max/1 -> Min/1, Sum1/1
  IC1/1 -> Sum/3
  Intake/1 -> Sum/2
  Constant/1 -> Max/1
  Demand/1 -> Unit Delay1/1
  Unit Delay1/1 -> Sum/1

== system Water_Supply_Network_AMONG_US/Well1 ==
  Constant : Constant  Value=Inf
  Out : Outport
  wires:
  Constant/1 -> Out/1

== system Water_Supply_Network_AMONG_US/Well2 ==
  Constant : Constant  Value=Inf
  availableWater : Outport
  wires:
  Constant/1 -> availableWater/1

== system Water_Supply_Network_AMONG_US/Well3 ==
  Constant : Constant  Value=Inf
  availableWater : Outport
  wires:
  Constant/1 -> availableWater/1

== system Water_Supply_Network_AMONG_US/Well4 ==
  Constant : Constant  Value=Inf
  availableWater : Outport
  wires:
  Constant/1 -> availableWater/1

== stateflow chart Water_Supply_Network_AMONG_US/Controller ==
  state Example2
    en:
    pumpSwitch = TRUE;
  state Example1
    en:
    pumpSwitch = FALSE;
  Example1 -> Example2 : [currentWater<maxWater]
  Example2 -> Example1 : [currentWater>=maxWater]
  (default) -> Example1
  data: currentWater input [0..]; maxWater input [0..]; pumpSwitch output boolean
